simulink model "boostObserver_complete"  (R2020a)
settings: Solver=ode45  StartTime=0.0  StopTime=1.2  FixedStep=0.0005  AbsTol=1e-06  EnableMultiTasking=on
InitFcn:
  | kp=0.01;
  | ki=0.01;
  | 
  | k=2;
  | em=100000000;
  | GE=1/em;
  | GU=k*ki/GE;
  | GCE=k*kp/GU;
model workspace (MAT data in the model file):
  time = 0.8
values from neighbouring files (symbols this model uses):
  AlarmDeadTime = 0.50    (= 0.5)    [BoostFaultSimulation.m]    (also in workspace_atual.mat; workspace_certo.mat)
  B1f = [200 0]    [workspace_atual.mat]    (also in workspace_certo.mat)
  B2f = [200 0]    [workspace_atual.mat]    (also in workspace_certo.mat)
  CiL = [0 1]    [workspace_atual.mat]    (also in workspace_certo.mat)
  CVc = [1 0]    [workspace_atual.mat]    (also in workspace_certo.mat)
  F_11 = -16.4    [workspace_atual.mat]    (also in workspace_certo.mat)
  F_12 = -4812476.87956    [workspace_atual.mat]    (also in workspace_certo.mat)
  F_21 = -3.50877192982    [workspace_atual.mat]    (also in workspace_certo.mat)
  F_22 = -2.00703596657    [workspace_atual.mat]    (also in workspace_certo.mat)
  FaultClass = 0    [BoostFaultSimulation.m]    (also in workspace_atual.mat = 1; workspace_certo.mat = 1)
  iLFaultSwitch = 0    [BoostFaultSimulation.m]    (also in workspace_atual.mat; workspace_certo.mat)
  iLFaultTime = 1.70    (= 1.7)    [BoostFaultSimulation.m]    (also in workspace_atual.mat; workspace_certo.mat)
  L_11 = -176809.798019    [workspace_atual.mat]    (also in workspace_certo.mat)
  L_12 = -66005538231.6    [workspace_atual.mat]    (also in workspace_certo.mat)
  L_21 = 0.0967961040176    [workspace_atual.mat]    (also in workspace_certo.mat)
  L_22 = 350.985265141    [workspace_atual.mat]    (also in workspace_certo.mat)
  Lnew1 = [0.000426144297292  -1.37628182296; -0.636691353583  10000.3869597]    [workspace_atual.mat]    (also in workspace_certo.mat = [0.00144628510103  0.00148492117427; 0.000288596381821  0.00)
  Lnew2 = [0.000454345330516  -0.588943865675; 0.999552025739  4999.94512306]    [workspace_atual.mat]    (also in workspace_certo.mat = [0.00251672143174  0.00251025627081; 6.60131109739e-05  6.53)
  Q_1 = [13715.5123667  1; 1  0]    [workspace_atual.mat]    (also in workspace_certo.mat)
  Q_2 = [1  0; 0.00750867981628  1]    [workspace_atual.mat]    (also in workspace_certo.mat)
  R = 0.1    [boostResults2Latex.m]    (also in workspace_atual.mat = 0.082; workspace_certo.mat = 0.082)
  ReconfigSwitch = 0    [BoostFaultSimulation.m]    (also in workspace_atual.mat; workspace_certo.mat)
  ReconfigTime = 1.707    [BoostFaultSimulation.m]    (also in workspace_atual.mat; workspace_certo.mat)
  SourceAddFactor = 0.10    (= 0.1)    [BoostFaultSimulation.m]    (also in workspace_atual.mat; workspace_certo.mat)
  SourceAddSwitch = 0    [BoostFaultSimulation.m]    (also in workspace_atual.mat; workspace_certo.mat)
  SourceRemoveFactor = 0.10    (= 0.1)    [BoostFaultSimulation.m]    (also in workspace_atual.mat; workspace_certo.mat)
  T_1 = [1 -13715.5123667]    [workspace_atual.mat]    (also in workspace_certo.mat)
  T_2 = [-0.00750867981628 1]    [workspace_atual.mat]    (also in workspace_certo.mat)
  Ts = 0.0001    [workspace_atual.mat]    (also in workspace_certo.mat)
  uf = 190    [workspace_atual.mat]    (also in workspace_certo.mat)
  VcFaultSwitch = 0    [BoostFaultSimulation.m]    (also in workspace_atual.mat; workspace_certo.mat)
  VcFaultTime = 1.70    (= 1.7)    [BoostFaultSimulation.m]    (also in workspace_atual.mat; workspace_certo.mat)
  xe = obj.boostConverter.equilibriumstate(ve)    [BoostController.m]    (also in workspace_atual.mat = [7.62509288104 380]; workspace_certo.mat = [7.62509288104 380])
undefined symbols (not defined in the file or in its folder): MAXnet, MINnet
libraries: PhdLibrary x38, neural x36, dspstat3 x4, powerlib x2, powerlib_meascontrol x2
(part 1 of 3)
settings Model: SimulationMode=accelerator  Creator=d13go  LastModifiedBy=d13go
settings SolverCC: MaxConsecutiveZCs=10000  ZeroCrossAlgorithm=Adaptive  DecoupledContinuousIntegration=on  MinimalZcImpactIntegration=on
settings DataIOCC: SaveFinalState=on  SaveState=on  LoggingToFile=on
settings OptimizationCC: DefaultParameterBehavior=Inlined  UseDivisionForNetSlopeComputation=on  GainParamInheritBuiltInType=on  UseFloatMulNetSlope=on  InlineInvariantSignals=on  EfficientFloat2IntCast=on  LifeSpan=1
settings DebuggingCC: ReadBeforeWriteMsg=DisableAll  WriteAfterWriteMsg=DisableAll  WriteAfterReadMsg=DisableAll  AlgebraicLoopMsg=error  MaxConsecutiveZCsMsg=warning  MaskedZcDiagnostic=none  IgnoredZcDiagnostic=none  MultiTaskDSMMsg=none  SFUnexpectedBacktrackingDiag=warning  SFNoUnconditionalDefaultTransitionDiag=warning  ArithmeticOperatorsInVariantConditions=warning
settings HardwareCC: ProdLongLongMode=on
settings ModelReferenceCC: UpdateModelReferenceTargets=IfOutOfDate
settings SFSimCC: SFSimEcho=off  SimUseLocalCustomCode=off  MATLABDynamicMemAlloc=off  CustomCodeUndefinedFunction=UseInterfaceOnly
settings RTWCC: GenerateReport=on  RTWUseLocalCustomCode=off  LaunchReport=on
settings CodeAppCC: ForceParamTrailComments=on
settings GRTTargetCC: TargetLangStandard=C89/C90 (ANSI)  CombineSignalStateStructs=on  MatFileLogging=off  SupportVariableSizeSignals=on
settings ConfigComp: CovMetricSettings=dw  CovHtmlReporting=on  CovSaveCumulativeToWorkspaceVar=on  CovSaveSingleToWorkspaceVar=on  CovExternalEMLEnable=off
settings SimscapeCC: SimscapeNormalizeSystem=off

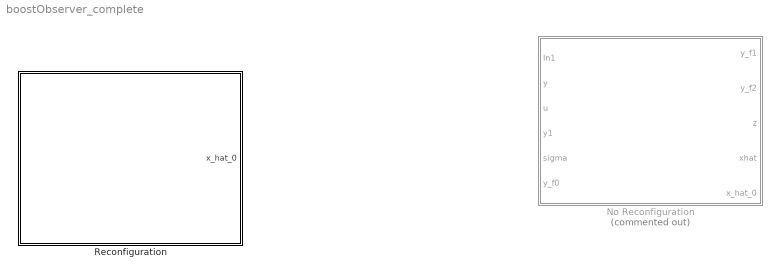
== system boostObserver_complete ==
  No Reconfiguration : Subsystem  Commented=on
  Reconfiguration : Subsystem

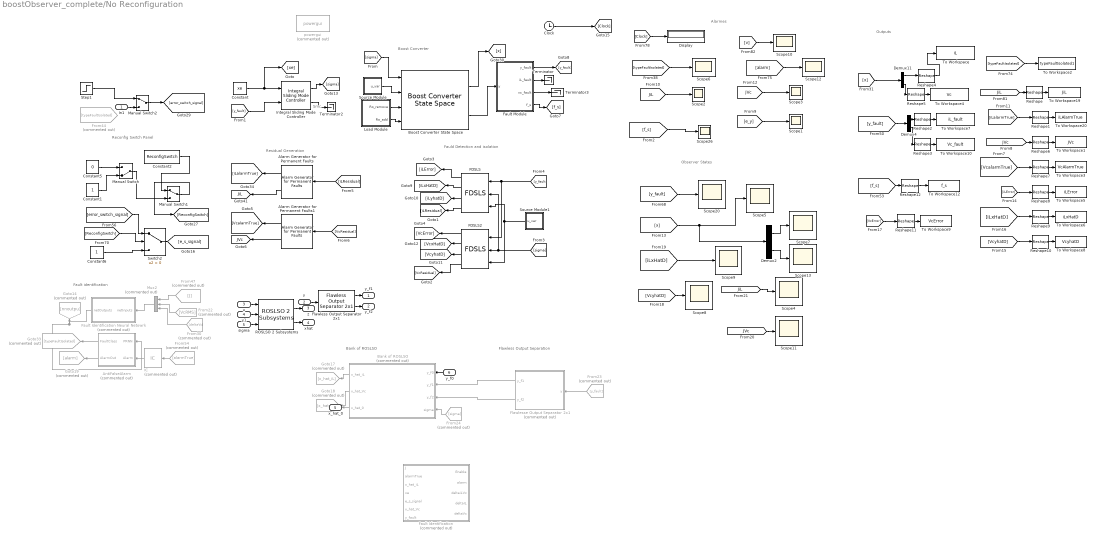
== system boostObserver_complete/No Reconfiguration ==
  note: Fauld Detection and isolation
  note: Smc
  note: Alarmes
  note: Observer States
  note: Residual Generation
  note: Boost Converter
  note: Outputs
  note: Reconfig Switch Panel
  note: Fault identification
  note: Bank of ROSLSO
  note: Flawless Output Separation
  In1 : Inport
  y : Inport  Port=2
  u : Inport  Port=3
  y1 : Inport  Port=4
  sigma : Inport  Port=5
  y_f0 : Inport  Port=6
  Alarm Generator for Permanent Faults : PhdLibrary/Alarm Generator for Permanent Faults  Jth=iLJth  r0=0
      settings: SourceProductName=Phd Diego
  Alarm Generator for Permanent Faults1 : PhdLibrary/Alarm Generator for Permanent Faults  Jth=iLJth  r0=0
      settings: SourceProductName=Phd Diego
  AntiFalseAlarm : Subsystem  Commented=on
  Bank of ROSLSO : Subsystem  Commented=on
  Boost Converter State Space : PhdLibrary/Boost Converter  State Space  A1=A1  A2=A2  B1=B1  R=R  Ro=Ro  Cmatrix=Cmatrix  c=c  LoadAddFactor=LoadAddFactor  LoadRemoveFactor=LoadRemoveFactor
      settings: SourceProductName=Phd Diego
  Clock : Clock
  Constant : Constant  Value=xe  VectorParams1D=off
  Constant1 : Constant
  Constant2 : Constant  Value=ReconfigSwitch
  Constant5 : Constant  Value=0
  Constant6 : Constant
  Demux11 : Demux  Outputs=2
  Demux2 : Demux  Outputs=2
  Demux4 : Demux  Outputs=2
  Display : Display
  FDSLS : PhdLibrary/FDSLS  A1=A1  A2=A2  B1=B1  B2=B2  L=Lnew1  yhat0=[0;0]  x0=[0;0]  Qr=[1 0]
      settings: SourceProductName=Phd Diego
  FDSLS2 : PhdLibrary/FDSLS  A1=A1  A2=A2  B1=B1  B2=B2  L=Lnew2  yhat0=[0;0]  x0=[0;0]  Qr=[0 1]
      settings: SourceProductName=Phd Diego
  Fault Identification : Subsystem  Commented=on
  Fault Identification Neural Netowrk : Subsystem  Commented=on
  Fault Module : Subsystem
  Flawless Output Separator 2x1 : PhdLibrary/Flawless Output  Separator 2x1  Cf1=0  Cf2=0
      settings: SourceProductName=Phd Diego
  Flawlesse Output Separator 2x1 : Subsystem  Commented=on  mask(Flawless Output Separator){Cf1=0, Cf2=0}
      mask prompts: Cf1 "Fault matrix 1"; Cf2 "Fault matrix 2"
      mask help: Separates the 2x1 output
  From22 : From  Commented=on  GotoTag=VcRMS  TagVisibility=global
  From23 : From  Commented=on  GotoTag=y_fault
  From24 : From  Commented=on  GotoTag=sigma
  From30 : From  Commented=on  GotoTag=deltaVc
  From44 : From  Commented=on  GotoTag=typeFaultIsolated
  From47 : From  Commented=on  GotoTag=J  TagVisibility=global
  From54 : From  Commented=on  GotoTag=alarmTrue
  Goto14 : Goto  Commented=on  GotoTag=nnoutpu
  Goto17 : Goto  Commented=on  GotoTag=x_hat_iL
  Goto18 : Goto  Commented=on  GotoTag=x_hat_Vc
  Goto19 : Goto  Commented=on  GotoTag=alarm
  Goto33 : Goto  Commented=on  GotoTag=typeFaultIsolated
  IC : InitialCondition  Commented=on  Value=0
  Integral Sliding Mode Controller : PhdLibrary/Integral Sliding  Mode Controller  KiVc=SmIntegralGain  KVc=SmVcGain  ueq=ueq  Smep=Smep  KiL=SmiLGain  Freq=SmFrequency  x0=0
      settings: SourceProductName=Phd Diego
  Load Module : Subsystem
  Manual Switch : ManualSwitch  CurrentSetting=0
  Manual Switch1 : ManualSwitch
  Manual Switch2 : ManualSwitch
  Mux2 : Mux  Commented=on  Inputs=3
  ROSLSO 2 Subsystems : PhdLibrary/ROSLSO  2 Subsystems  B1=0  B2=0  T=0  F1=0  F2=0  L1=0  L2=0  Q=0  z0=0
      settings: SourceProductName=Phd Diego
  Reshape{,1..12} (13 alike) : Reshape
  Scope{1..13,20,26} (15 alike) : Scope
  Source Module : Subsystem
  Source Module1 : Subsystem
  Step1 : Step  Time=ReconfigTime  After=FaultClass  SampleTime=0
  Switch2 : Switch  Criteria=u2 > Threshold
  Terminator : Terminator
  Terminator2 : Terminator
  Terminator3 : Terminator
  To Workspace : ToWorkspace  VariableName=iL  SaveFormat=Timeseries  SampleTime=-1
  To Workspace1 : ToWorkspace  VariableName=JVc  SaveFormat=Timeseries  SampleTime=-1
  To Workspace10 : ToWorkspace  VariableName=Vc_fault  SaveFormat=Timeseries  SampleTime=-1
  To Workspace12 : ToWorkspace  VariableName=f_s  SaveFormat=Timeseries  SampleTime=-1
  To Workspace19 : ToWorkspace  VariableName=JiL  SaveFormat=Timeseries  SampleTime=-1
  To Workspace2 : ToWorkspace  VariableName=typeFaultIsolated1  SaveFormat=Timeseries  SampleTime=-1
  To Workspace20 : ToWorkspace  VariableName=iLAlarmTrue  SaveFormat=Timeseries  SampleTime=-1
  To Workspace3 : ToWorkspace  VariableName=VcAlarmTrue  SaveFormat=Timeseries  SampleTime=-1
  To Workspace4 : ToWorkspace  VariableName=Vc  SaveFormat=Timeseries  SampleTime=-1
  To Workspace5 : ToWorkspace  VariableName=iLError  SaveFormat=Timeseries  SampleTime=-1
  To Workspace6 : ToWorkspace  VariableName=iLxHatD  SaveFormat=Timeseries  SampleTime=-1
  To Workspace7 : ToWorkspace  VariableName=iL_fault  SaveFormat=Timeseries  SampleTime=-1
  To Workspace8 : ToWorkspace  VariableName=VcyhatD  SaveFormat=Timeseries  SampleTime=-1
  To Workspace9 : ToWorkspace  VariableName=VcError  SaveFormat=Timeseries  SampleTime=-1
  powergui : powerlib/powergui  Priority=1  Commented=on  SimulationMode=Discrete  SampleTime=50e-6  frequency=60  Iterations=50  frequencyindice=0  Pbase=100e6  ErrMax=1e-4  UnitsV=kV  UnitsW=MW  buscounter=0  FunctionMessages=off  echomessages=off  EnableUseOfTLC=off  CurrentSourceSwitches=off  DisableSnubberDevices=off  DisableRonSwitches=off  DisableVfSwitches=off  DisplayEquations=off  AutomaticDiscreteSolvers=off  SolverType=Tustin/Backward Euler (TBE)  Interpol=off  ExternalGateDelay=off  methode=off  Ts=100  x0status=blocks  SPID=on  SwTol=0  HookPort=off  NonlinearTolerance=1e-4  nMaxIteration=100  ContinueOnMaxIteration=off  RestoreLinks=warning  ResistiveCurrentMeasurement=off  Frange=[0:2:500]  Ylog=off  Xlog=on  ShowGrid=off  save=off  variable=ZData  structure=0  ZoomFFT=off  StartTime=0.0  cycles=1  DisplayStyle=1  fundamental=60  FreqAxis=off  MaxFrequency=1000  frequencyindicesteady=1  RmsSteady=1  display=off
  y_f1 : Outport
  y_f2 : Outport  Port=2
  z : Outport  Port=3
  xhat : Outport  Port=4
  x_hat_0 : Outport  Port=5
  tag scope: JVc=global, JiL=global
  wires:
  FDSLS2/1 -> [VcError]
  FDSLS/2 -> [iLxHatD]
  [sigma] -> FDSLS2/2, FDSLS/2
  [iLalarmTrue] -> Reshape1/1
  Reshape11/1 -> To Workspace9/1
  [sigma] -> Boost Converter State Space/1
  Demux2/1 -> Scope7/1
  Reshape9/1 -> To Workspace6/1
  [VcalarmTrue] -> Reshape7/1
  Reshape2/1 -> To Workspace7/1
  [x] -> Demux2/1, Scope5/1
  Load Module/2(Ro_add) -> Boost Converter State Space/4
  Constant/1 -> [xe], Integral Sliding Mode Controller/1
  Constant5/1 -> Manual Switch/1
  [VcyhatD] -> Reshape10/1
  Reshape/1 -> To Workspace19/1
  Reshape4/1 -> To Workspace/1
  Clock/1 -> [Clock]
  [VcResidual] -> Alarm Generator for Permanent Faults1/1
  Alarm Generator for Permanent Faults1/1 -> [VcalarmTrue]
  Reshape10/1 -> To Workspace8/1
  Fault Module/1(y_fault) -> [y_fault]
  [x] -> Demux11/1
  Demux4/1 -> Reshape2/1
  y_f0/1 -> Bank of ROSLSO/1(y_f0)
  Demux11/1 -> Reshape4/1
  FDSLS/4 -> [iLResidual]
  Integral Sliding Mode Controller/2 -> Terminator2/1
  Reshape8/1 -> To Workspace5/1
  Fault Module/3(vc_fault) -> Terminator3/1
  FDSLS/3 -> [iLyhatD]
  Reshape5/1 -> To Workspace4/1
  [JiL] -> Reshape/1
  FDSLS2/4 -> [VcResidual]
  [y_fault] -> Scope20/1
  Boost Converter State Space/2 -> Fault Module/1(y)
  [y_fault] -> FDSLS2/1, FDSLS/1
  [typeFaultIsolated] -> To Workspace2/1
  [f_s] -> Scope26/1
  Reshape1/1 -> To Workspace20/1
  [e_y] -> Scope1/1
  FDSLS2/3 -> [VcyhatD]
  [y_fault] -> Demux4/1
  [error_switch_signal] -> Switch2/1
  [Clock] -> Display/1
  Demux2/2 -> Scope13/1
  Boost Converter State Space/1 -> [x]
  [v] -> Scope10/1
  [JiL] -> Scope2/1
  [JVc] -> Scope3/1
  Alarm Generator for Permanent Faults/2 -> [JiL]
  [alarm] -> Scope12/1
  [VcError] -> Reshape11/1
  Integral Sliding Mode Controller/1 -> [sigma]
  Alarm Generator for Permanent Faults1/2 -> [JVc]
  [iLxHatD] -> Reshape9/1
  [typeFaultIsolated] -> Scope6/1
  [JVc] -> Reshape6/1
  Bank of ROSLSO/3(x_hat_0) -> x_hat_0/1
  [iLResidual] -> Alarm Generator for Permanent Faults/1
  [f_s] -> Reshape12/1
  Load Module/1(Ro_remove) -> Boost Converter State Space/3
  Demux4/2 -> Reshape3/1
  [iLError] -> Reshape8/1
  Step1/1 -> Manual Switch2/1
  FDSLS/1 -> [iLError]
  Reshape6/1 -> To Workspace1/1
  Demux11/2 -> Reshape5/1
  Switch2/1 -> [e_s_signal]
  Alarm Generator for Permanent Faults/1 -> [iLalarmTrue]
  Source Module1/1(u_var) -> FDSLS2/3, FDSLS/3
  [iLxHatD] -> Scope9/1
  Source Module/1(u_var) -> Boost Converter State Space/2
  FDSLS2/2 -> [VcxHatD]
  Fault Module/2(iL_fault) -> Terminator/1
  [JVc] -> Scope11/1
  Reshape3/1 -> To Workspace10/1
  Reshape7/1 -> To Workspace3/1
  Reshape12/1 -> To Workspace12/1
  [JiL] -> Scope4/1
  [VcyhatD] -> Scope8/1
  [y_fault] -> Integral Sliding Mode Controller/2
  Bank of ROSLSO/1(x_hat_iL) -> Goto17/1
  Manual Switch2/1 -> [error_switch_signal]
  Constant1/1 -> Manual Switch/2
  Constant2/1 -> Manual Switch1/1
  Manual Switch/1 -> Manual Switch1/2
  [ReconfigSwitch] -> Switch2/2
  Manual Switch1/1 -> [ReconfigSwitch]
  Constant6/1 -> Switch2/3
  Fault Module/4(f_s) -> [f_s]
  Fault Identification Neural Netowrk/1(netOutputs) -> AntiFalseAlarm/1(PRNN), Goto14/1
  From30/1 -> Mux2/3
  IC/1 -> AntiFalseAlarm/2(Alarm)
  From54/1 -> IC/1
  AntiFalseAlarm/1(FaultClass) -> Goto33/1
  Mux2/1 -> Fault Identification Neural Netowrk/1(netInputs)
  AntiFalseAlarm/2(AlarmOut) -> Goto19/1
  From47/1 -> Mux2/1
  From22/1 -> Mux2/2
  Flawlesse Output Separator 2x1/1(y_f1) -> Bank of ROSLSO/2(y_f1)
  From23/1 -> Flawlesse Output Separator 2x1/1(y)
  Bank of ROSLSO/2(x_hat_Vc) -> Goto18/1
  From24/1 -> Bank of ROSLSO/4(sigma)
  Flawlesse Output Separator 2x1/2(y_f2) -> Bank of ROSLSO/3(y_f2)
  u/1 -> ROSLSO 2 Subsystems/1
  ROSLSO 2 Subsystems/1 -> z/1
  y1/1 -> ROSLSO 2 Subsystems/2
  In1/1 -> Manual Switch2/2
  sigma/1 -> ROSLSO 2 Subsystems/3
  ROSLSO 2 Subsystems/2 -> xhat/1
  Flawless Output Separator 2x1/2 -> y_f2/1
  y/1 -> Flawless Output Separator 2x1/1
  Flawless Output Separator 2x1/1 -> y_f1/1

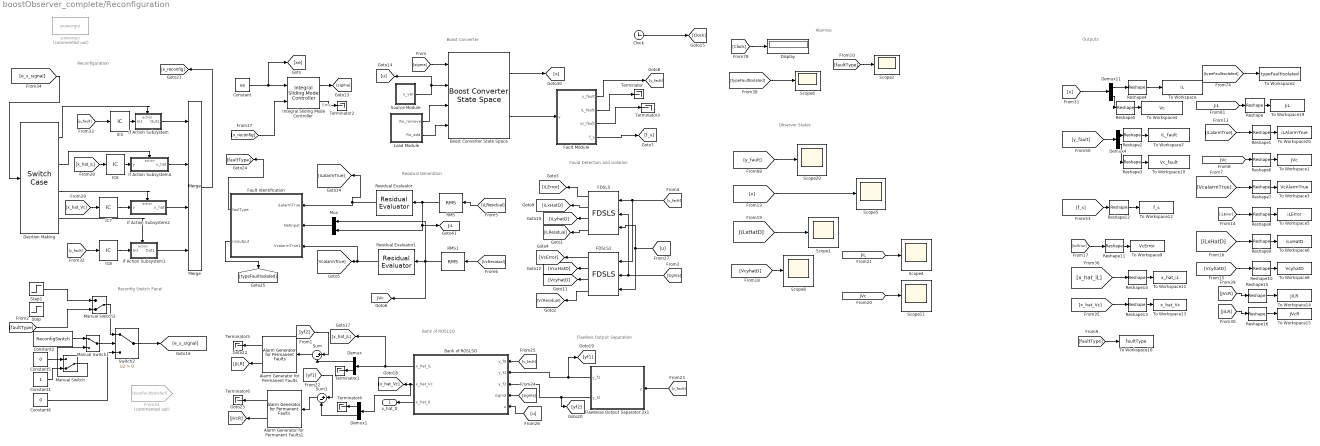
== system boostObserver_complete/Reconfiguration ==
  note: Fauld Detection and isolation
  note: Smc
  note: Alarmes
  note: Observer States
  note: Residual Generation
  note: Boost Converter
  note: Outputs
  note: Bank of ROSLSO
  note: Flawless Output Separation
  note: Reconfiguration
  note: Reconfig Switch Panel
  Alarm Generator for Permanent Faults : PhdLibrary/Alarm Generator for Permanent Faults  Jth=0  r0=0
      settings: SourceProductName=Phd Diego
  Alarm Generator for Permanent Faults1 : PhdLibrary/Alarm Generator for Permanent Faults  Jth=0  r0=0
      settings: SourceProductName=Phd Diego
  Bank of ROSLSO : Subsystem
  Boost Converter State Space : PhdLibrary/Boost Converter  State Space  A1=A1  A2=A2  B1=B1  R=R  Ro=Ro  Cmatrix=Cmatrix  c=c  LoadAddFactor=LoadAddFactor  LoadRemoveFactor=LoadRemoveFactor
      settings: SourceProductName=Phd Diego
  Clock : Clock
  Constant : Constant  Value=xe  VectorParams1D=off
  Constant1 : Constant
  Constant2 : Constant  Value=ReconfigSwitch
  Constant5 : Constant  Value=0
  Constant6 : Constant  Value=0
  Decition Making : SwitchCase  CaseConditions={[0],[1],[2]}
  Demux{,1,4,11} (4 alike) : Demux  Outputs=2
  Display : Display
  FDSLS : PhdLibrary/FDSLS  A1=A1  A2=A2  B1=B1  B2=B2  L=Lnew1  yhat0=[0;0]  x0=[0;0]  Qr=[1 0]
      settings: SourceProductName=Phd Diego
  FDSLS2 : PhdLibrary/FDSLS  A1=A1  A2=A2  B1=B1  B2=B2  L=Lnew2  yhat0=[0;0]  x0=[0;0]  Qr=[0 1]
      settings: SourceProductName=Phd Diego
  Fault Identification : Subsystem
  Fault Module : Subsystem
  Flawlesse Output Separator 2x1 : Subsystem  mask(Flawless Output Separator){Cf1=CiL, Cf2=CVc}
      mask prompts: Cf1 "Fault matrix 1"; Cf2 "Fault matrix 2"
      mask help: Separates the 2x1 output
  From44 : From  Commented=on  GotoTag=typeFaultIsolated
  IC{5..8} (4 alike) : InitialCondition  Value=[0;0]
  If Action Subsystem : Subsystem  TreatAsAtomicUnit=on
  If Action Subsystem1 : Subsystem  TreatAsAtomicUnit=on
  If Action Subsystem2 : Subsystem  TreatAsAtomicUnit=on
  If Action Subsystem4 : Subsystem  TreatAsAtomicUnit=on
  Integral Sliding Mode Controller : PhdLibrary/Integral Sliding  Mode Controller  KiVc=SmIntegralGain  KVc=SmVcGain  ueq=ueq  Smep=Smep  KiL=SmiLGain  Freq=7000  x0=[0;0]  Ts=0
      settings: SourceProductName=Phd Diego
  Load Module : Subsystem
  Manual Switch : ManualSwitch  CurrentSetting=0
  Manual Switch1 : ManualSwitch
  Manual Switch2 : ManualSwitch  CurrentSetting=0
  Merge : Merge  Inputs=4
  Mux : Mux  Inputs=2
  RMS : powerlib_meascontrol/Measurements/RMS  TrueRMS=on  Freq=RMSfrequency  RMSInit=0  Ts=Ts
  RMS1 : powerlib_meascontrol/Measurements/RMS  TrueRMS=on  Freq=RMSfrequency  RMSInit=0  Ts=Ts
  Reshape{,1..16} (17 alike) : Reshape
  Residual Evaluator : PhdLibrary/Residual Evaluator  Jth=iLJth
      settings: SourceProductName=Phd Diego
  Residual Evaluator1 : PhdLibrary/Residual Evaluator  Jth=VcJth
      settings: SourceProductName=Phd Diego
  Scope{1..2,4..6,8,11,20} (8 alike) : Scope
  Source Module : Subsystem
  Step : Step  Time=1.707  After=2  SampleTime=0
  Step1 : Step  Time=ReconfigTime  After=FaultClass  SampleTime=0
  Sum : Sum  Inputs=|+-
  Sum1 : Sum  Inputs=|+-
  Switch2 : Switch  Criteria=u2 > Threshold
  Terminator{,1..6} (7 alike) : Terminator
  To Workspace : ToWorkspace  VariableName=iL  SaveFormat=Timeseries  SampleTime=-1
  To Workspace1 : ToWorkspace  VariableName=JVc  SaveFormat=Timeseries  SampleTime=-1
  To Workspace10 : ToWorkspace  VariableName=Vc_fault  SaveFormat=Timeseries  SampleTime=-1
  To Workspace11 : ToWorkspace  VariableName=x_hat_iL  SaveFormat=Timeseries  SampleTime=-1
  To Workspace12 : ToWorkspace  VariableName=f_s  SaveFormat=Timeseries  SampleTime=-1
  To Workspace13 : ToWorkspace  VariableName=x_hat_Vc  SaveFormat=Timeseries  SampleTime=-1
  To Workspace14 : ToWorkspace  VariableName=JiLR  SaveFormat=Timeseries  SampleTime=-1
  To Workspace15 : ToWorkspace  VariableName=JVcR  SaveFormat=Timeseries  SampleTime=-1
  To Workspace16 : ToWorkspace  VariableName=faultType  SaveFormat=Timeseries  SampleTime=-1
  To Workspace19 : ToWorkspace  VariableName=JiL  SaveFormat=Timeseries  SampleTime=-1
  To Workspace2 : ToWorkspace  VariableName=typeFaultIsolated  SaveFormat=Timeseries  SampleTime=-1
  To Workspace20 : ToWorkspace  VariableName=iLAlarmTrue  SaveFormat=Timeseries  SampleTime=-1
  To Workspace3 : ToWorkspace  VariableName=VcAlarmTrue  SaveFormat=Timeseries  SampleTime=-1
  To Workspace4 : ToWorkspace  VariableName=Vc  SaveFormat=Timeseries  SampleTime=-1
  To Workspace5 : ToWorkspace  VariableName=iLError  SaveFormat=Timeseries  SampleTime=-1
  To Workspace6 : ToWorkspace  VariableName=iLxHatD  SaveFormat=Timeseries  SampleTime=-1
  To Workspace7 : ToWorkspace  VariableName=iL_fault  SaveFormat=Timeseries  SampleTime=-1
  To Workspace8 : ToWorkspace  VariableName=VcyhatD  SaveFormat=Timeseries  SampleTime=-1
  To Workspace9 : ToWorkspace  VariableName=VcError  SaveFormat=Timeseries  SampleTime=-1
  powergui : powerlib/powergui  Priority=1  Commented=on  SimulationMode=Discrete  SampleTime=50e-6  frequency=60  Iterations=50  frequencyindice=0  Pbase=100e6  ErrMax=1e-4  UnitsV=kV  UnitsW=MW  buscounter=0  FunctionMessages=off  echomessages=off  EnableUseOfTLC=off  CurrentSourceSwitches=off  DisableSnubberDevices=off  DisableRonSwitches=off  DisableVfSwitches=off  DisplayEquations=off  AutomaticDiscreteSolvers=off  SolverType=Tustin/Backward Euler (TBE)  Interpol=off  ExternalGateDelay=off  methode=off  Ts=100  x0status=blocks  SPID=on  SwTol=0  HookPort=off  NonlinearTolerance=1e-4  nMaxIteration=100  ContinueOnMaxIteration=off  RestoreLinks=warning  ResistiveCurrentMeasurement=off  Frange=[0:2:500]  Ylog=off  Xlog=on  ShowGrid=off  save=off  variable=ZData  structure=0  ZoomFFT=off  StartTime=0.0  cycles=1  DisplayStyle=1  fundamental=60  FreqAxis=off  MaxFrequency=1000  frequencyindicesteady=1  RmsSteady=1  display=off
  x_hat_0 : Outport
  tag scope: JVc=global, JiL=global
  wires:
  FDSLS2/1 -> [VcError]
  FDSLS/2 -> [iLxHatD]
  [sigma] -> FDSLS2/2, FDSLS/2
  [iLalarmTrue] -> Reshape1/1
  Reshape11/1 -> To Workspace9/1
  [sigma] -> Boost Converter State Space/1
  Reshape9/1 -> To Workspace6/1
  [VcalarmTrue] -> Reshape7/1
  Reshape2/1 -> To Workspace7/1
  [x] -> Scope5/1
  Constant/1 -> Integral Sliding Mode Controller/1, [xe]
  [VcyhatD] -> Reshape10/1
  Reshape/1 -> To Workspace19/1
  Reshape4/1 -> To Workspace/1
  Clock/1 -> [Clock]
  Residual Evaluator1/1 -> Fault Identification/3(VcalarmTrue1), [VcalarmTrue]
  Reshape10/1 -> To Workspace8/1
  Fault Module/1(y_fault) -> [y_fault]
  [x] -> Demux11/1
  Demux4/1 -> Reshape2/1
  [y_fault] -> Bank of ROSLSO/1(y_f0)
  Demux11/1 -> Reshape4/1
  FDSLS/4 -> [iLResidual]
  Integral Sliding Mode Controller/2 -> Terminator2/1
  Reshape8/1 -> To Workspace5/1
  Fault Module/3(vc_fault) -> Terminator3/1
  FDSLS/3 -> [iLyhatD]
  Reshape5/1 -> To Workspace4/1
  [JiL] -> Reshape/1
  FDSLS2/4 -> [VcResidual]
  [y_fault] -> Scope20/1
  Boost Converter State Space/2 -> Fault Module/1(y)
  [y_fault] -> FDSLS2/1, FDSLS/1
  [typeFaultIsolated] -> To Workspace2/1
  Reshape1/1 -> To Workspace20/1
  FDSLS2/3 -> [VcyhatD]
  [y_fault] -> Demux4/1
  [Clock] -> Display/1
  Boost Converter State Space/1 -> [x]
  [VcError] -> Reshape11/1
  Integral Sliding Mode Controller/1 -> [sigma]
  [iLxHatD] -> Reshape9/1
  [typeFaultIsolated] -> Scope6/1
  [JVc] -> Reshape6/1
  Bank of ROSLSO/3(x_hat_0) -> x_hat_0/1
  [f_s] -> Reshape12/1
  Demux4/2 -> Reshape3/1
  [iLError] -> Reshape8/1
  FDSLS/1 -> [iLError]
  Reshape6/1 -> To Workspace1/1
  Demux11/2 -> Reshape5/1
  Residual Evaluator/1 -> Fault Identification/1(iLalarmTrue), [iLalarmTrue]
  [u] -> FDSLS/3, FDSLS2/3
  [iLxHatD] -> Scope1/1
  FDSLS2/2 -> [VcxHatD]
  Fault Module/2(iL_fault) -> Terminator/1
  [JVc] -> Scope11/1
  Reshape3/1 -> To Workspace10/1
  Reshape7/1 -> To Workspace3/1
  Reshape12/1 -> To Workspace12/1
  [VcyhatD] -> Scope8/1
  Bank of ROSLSO/1(x_hat_iL) -> [x_hat_iL], Demux/1
  Fault Module/4(f_s) -> [f_s]
  [y_fault] -> Flawlesse Output Separator 2x1/1(y)
  [sigma] -> Bank of ROSLSO/4(sigma)
  Flawlesse Output Separator 2x1/2(y_f2) -> [yf2], Bank of ROSLSO/3(y_f2)
  [u] -> Bank of ROSLSO/5(u)
  [x_hat_Vc] -> IC7/1
  [e_s_signal] -> Decition Making/1
  If Action Subsystem2/1(x_hat) -> Merge/3
  IC8/1 -> If Action Subsystem1/1(In1)
  IC6/1 -> If Action Subsystem4/1(y)
  [x_hat_iL] -> IC6/1
  Merge/1 -> [x_reconfig]
  IC5/1 -> If Action Subsystem/1(In1)
  If Action Subsystem1/1(Out1) -> Merge/4
  Decition Making/2 -> If Action Subsystem4/Action
  Decition Making/1 -> If Action Subsystem/Action
  Decition Making/3 -> If Action Subsystem2/Action
  IC7/1 -> If Action Subsystem2/1(y)
  [y_fault] -> IC5/1
  Decition Making/4 -> If Action Subsystem1/Action
  If Action Subsystem4/1(x_hat) -> Merge/2
  [y_fault] -> IC8/1
  If Action Subsystem/1(Out1) -> Merge/1
  [x_hat_iL] -> Reshape14/1
  Reshape13/1 -> To Workspace13/1
  [x_hat_Vc] -> Reshape13/1
  Reshape14/1 -> To Workspace11/1
  Step1/1 -> Manual Switch2/1
  Manual Switch/1 -> Manual Switch1/2
  Constant2/1 -> Manual Switch1/1
  Constant1/1 -> Manual Switch/2
  Constant5/1 -> Manual Switch/1
  Manual Switch1/1 -> Switch2/2
  Constant6/1 -> Switch2/3
  Manual Switch2/1 -> Switch2/1
  Switch2/1 -> [e_s_signal]
  Source Module/1(u_var) -> Boost Converter State Space/2, [u]
  Bank of ROSLSO/2(x_hat_Vc) -> Demux1/1, [x_hat_Vc]
  Flawlesse Output Separator 2x1/1(y_f1) -> [yf1], Bank of ROSLSO/2(y_f1)
  [yf2] -> Sum/1
  Alarm Generator for Permanent Faults/2 -> [JiLR]
  Demux/1 -> Sum/2
  [yf1] -> Sum1/1
  Demux1/2 -> Sum1/2
  Sum1/1 -> Alarm Generator for Permanent Faults1/1
  [JVcR] -> Reshape15/1
  [JiLR] -> Reshape16/1
  Reshape15/1 -> To Workspace14/1
  Reshape16/1 -> To Workspace15/1
  [JiL] -> Scope4/1
  Alarm Generator for Permanent Faults1/2 -> [JVcR]
  Sum/1 -> Alarm Generator for Permanent Faults/1
  Demux/2 -> Terminator1/1
  Demux1/1 -> Terminator4/1
  Alarm Generator for Permanent Faults/1 -> Terminator5/1
  Alarm Generator for Permanent Faults1/1 -> Terminator6/1
  [x_reconfig] -> Integral Sliding Mode Controller/2
  RMS/1 -> [JiL], Mux/2, Residual Evaluator/1
  [VcResidual] -> RMS1/1
  Load Module/2(Ro_add) -> Boost Converter State Space/4
  Load Module/1(Ro_remove) -> Boost Converter State Space/3
  Mux/1 -> Fault Identification/2(Netinput)
  Fault Identification/1(faulType) -> [faultType]
  Fault Identification/2(nnoutput) -> [typeFaultIsolated]
  [faultType] -> Manual Switch2/2
  [faultType] -> To Workspace16/1
  [faultType] -> Scope2/1
  [iLResidual] -> RMS/1
  RMS1/1 -> Mux/1, [JVc], Residual Evaluator1/1

== system boostObserver_complete/No Reconfiguration/AntiFalseAlarm ==
  PRNN : Inport
  Alarm : Inport  Port=2
  Constant7 : Constant
  FaultDetecition1 : Switch  Criteria=u2 > Threshold
  Product1 : Product
  Step1 : Step  Time=AlarmDeadTime  SampleTime=0
  FaultClass : Outport
  AlarmOut : Outport  Port=2
  wires:
  PRNN/1 -> FaultDetecition1/1
  Constant7/1 -> FaultDetecition1/3
  Step1/1 -> Product1/1
  Alarm/1 -> Product1/2
  FaultDetecition1/1 -> FaultClass/1
  Product1/1 -> AlarmOut/1, FaultDetecition1/2

== system boostObserver_complete/No Reconfiguration/Bank of ROSLSO ==
  y_f0 : Inport
  y_f1 : Inport  Port=2
  y_f2 : Inport  Port=3
  sigma : Inport  Port=4
  Constant : Constant  Value=uf  VectorParams1D=off
  ROSLSO 2 Subsystems : Subsystem  mask(ROSLSO){B1=B1f, B2=B2f, T=T_1, F1=F_11, F2=F_12, L1=L_11, L2=L_12, Q=Q_1, z0=0}
      mask prompts: B1 "Input matrix system 1:"; B2 "Input matrix system 2:"; T "Input gain matrix:"; F1 "Observer matrix system 1:"; F2 "Observer matrix system 2:"; L1 "Output gain matrix system 1:"; L2 "Output gain matrix system 2:"; Q "Weight matrix"; z0 "Initial conditions:"
      mask help:
      | Reduced Order Switched Linear Systems Observer
      | Estimates only the unmensured variables and concatenate with output
  ROSLSO 2 Subsystems1 : Subsystem  mask(ROSLSO){B1=B1f, B2=B2f, T=T_2, F1=F_21, F2=F_22, L1=L_21, L2=L_22, Q=Q_2, z0=0}
      mask prompts: B1 "Input matrix system 1:"; B2 "Input matrix system 2:"; T "Input gain matrix:"; F1 "Observer matrix system 1:"; F2 "Observer matrix system 2:"; L1 "Output gain matrix system 1:"; L2 "Output gain matrix system 2:"; Q "Weight matrix"; z0 "Initial conditions:"
      mask help:
      | Reduced Order Switched Linear Systems Observer
      | Estimates only the unmensured variables and concatenate with output
  Terminator : Terminator
  Terminator1 : Terminator
  x_hat_iL : Outport
  x_hat_Vc : Outport  Port=2
  x_hat_0 : Outport  Port=3
  wires:
  sigma/1 -> ROSLSO 2 Subsystems/3(sigma), ROSLSO 2 Subsystems1/3(sigma)
  y_f1/1 -> ROSLSO 2 Subsystems/2(y)
  y_f2/1 -> ROSLSO 2 Subsystems1/2(y)
  Constant/1 -> ROSLSO 2 Subsystems/1(u), ROSLSO 2 Subsystems1/1(u)
  ROSLSO 2 Subsystems1/2(xhat) -> x_hat_Vc/1
  ROSLSO 2 Subsystems/2(xhat) -> x_hat_iL/1
  ROSLSO 2 Subsystems/1(z) -> Terminator/1
  ROSLSO 2 Subsystems1/1(z) -> Terminator1/1
  y_f0/1 -> x_hat_0/1

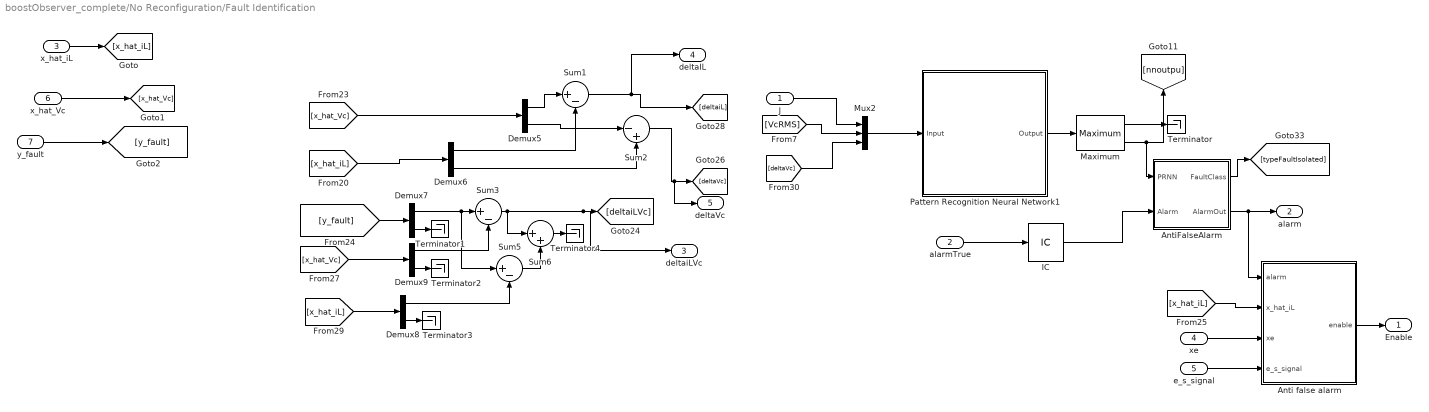
== system boostObserver_complete/No Reconfiguration/Fault Identification ==
  J : Inport
  alarmTrue : Inport  Port=2
  x_hat_iL : Inport  Port=3
  xe : Inport  Port=4
  e_s_signal : Inport  Port=5
  x_hat_Vc : Inport  Port=6
  y_fault : Inport  Port=7
  Anti false alarm : Subsystem
  AntiFalseAlarm : Subsystem
  Demux{5..9} (5 alike) : Demux  Outputs=2
  IC : InitialCondition  Value=0
  Maximum : dspstat3/Maximum  operation=maximum  fcn=Value and Index  indexBase=One  operateOver=Each column  Dimension=1  InputProcessing=Columns as channels (frame based)  reset=None  roiEnable=off  roiType=Rectangles  roiPortion=Entire ROI  roiOutput=Individual statistics for each ROI  roiFlag=off  roundingMode=Floor  overflowMode=off  accumDataTypeStr=Inherit: Same as product output  accumLastDataTypeStr=Inherit: Same as product output
  Mux2 : Mux  Inputs=3
  Pattern Recognition Neural Network1 : Subsystem
      mask help: Pattern Recognition Neural Network
      mask Display: e = 0.06;c1 = [120 150 230]/255;c2 = ([120 150 230]+0)/383;c3 = ([120 150 230]+128)/383;patch([0 1 1 0],[0 0 1 1],c1);patch([0 1 1 1-e 1-e 0+e],[0 0 1 1-e 0+e 0+e],c2);patch([0 0 1 1-e 0+e 0+e],[0 1 1 1-e 1-e 0+e],c3);plot([0 1 1 0 0],[0 0 1 1 0]);fprintf('NNET');port_label('input',1,' Input');port_label('output',1,'Output ');
  Sum1 : Sum  Inputs=|+-
  Sum2 : Sum  Inputs=|-+
  Sum3 : Sum  Inputs=|+-
  Sum5 : Sum  Inputs=|+-
  Sum6 : Sum  Inputs=|++
  Terminator{,1..4} (5 alike) : Terminator
  Enable : Outport
  alarm : Outport  Port=2
  deltaiLVc : Outport  Port=3
  deltaIL : Outport  Port=4
  deltaVc : Outport  Port=5
  wires:
  Demux6/2 -> Sum2/2
  Sum2/1 -> deltaVc/1, [deltaVc]
  Demux7/2 -> Terminator1/1
  Sum5/1 -> Sum6/2
  [y_fault] -> Demux7/1
  Sum3/1 -> deltaiLVc/1, [deltaiLVc], Sum6/1
  Demux5/2 -> Sum2/1
  [x_hat_Vc] -> Demux9/1
  Demux5/1 -> Sum1/1
  Demux9/1 -> Sum3/2
  [deltaVc] -> Mux2/3
  [x_hat_Vc] -> Demux5/1
  Demux6/1 -> Sum1/2
  Demux8/1 -> Sum5/2
  Demux7/1 -> Sum5/1, Sum3/1
  [VcRMS] -> Mux2/2
  [x_hat_iL] -> Demux6/1
  Sum1/1 -> deltaIL/1, [deltaiL]
  [x_hat_iL] -> Demux8/1
  Demux9/2 -> Terminator2/1
  Demux8/2 -> Terminator3/1
  J/1 -> Mux2/1
  Maximum/1 -> Terminator/1
  Pattern Recognition Neural Network1/1(Output) -> Maximum/1
  Mux2/1 -> Pattern Recognition Neural Network1/1(Input)
  Maximum/2 -> AntiFalseAlarm/1(PRNN), [nnoutpu]
  alarmTrue/1 -> IC/1
  IC/1 -> AntiFalseAlarm/2(Alarm)
  AntiFalseAlarm/1(FaultClass) -> [typeFaultIsolated]
  AntiFalseAlarm/2(AlarmOut) -> alarm/1, Anti false alarm/1(alarm)
  xe/1 -> Anti false alarm/3(xe)
  e_s_signal/1 -> Anti false alarm/4(e_s_signal)
  Anti false alarm/1(enable) -> Enable/1
  x_hat_iL/1 -> [x_hat_iL]
  [x_hat_iL] -> Anti false alarm/2(x_hat_iL)
  x_hat_Vc/1 -> [x_hat_Vc]
  y_fault/1 -> [y_fault]
  Sum6/1 -> Terminator4/1

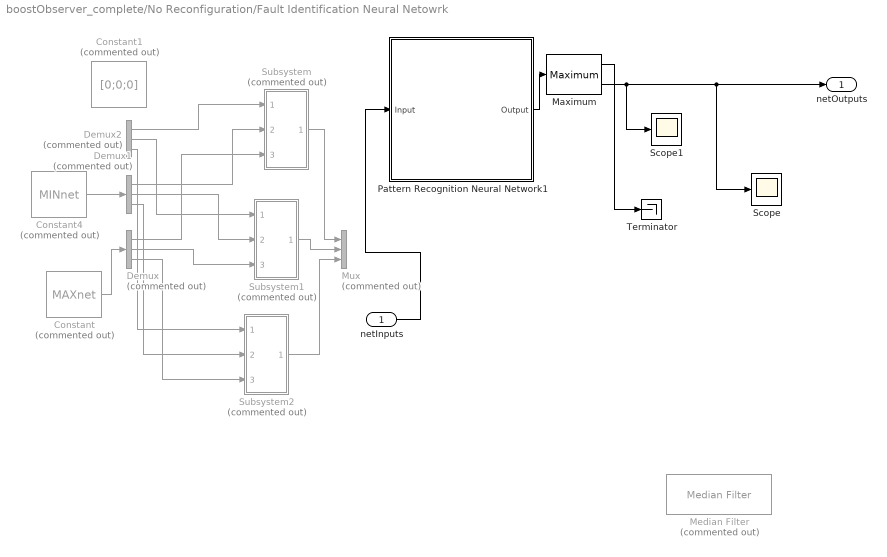
== system boostObserver_complete/No Reconfiguration/Fault Identification Neural Netowrk ==
  netInputs : Inport
  Constant : Constant  Commented=on  Value=MAXnet
  Constant1 : Constant  Commented=on  Value=[0;0;0]
  Constant4 : Constant  Commented=on  Value=MINnet
  Demux : Demux  Commented=on  Outputs=3
  Demux1 : Demux  Commented=on  Outputs=3
  Demux2 : Demux  Commented=on  Outputs=3
  Maximum : dspstat3/Maximum  operation=maximum  fcn=Value and Index  indexBase=One  operateOver=Each column  Dimension=1  InputProcessing=Columns as channels (frame based)  reset=None  roiEnable=off  roiType=Rectangles  roiPortion=Entire ROI  roiOutput=Individual statistics for each ROI  roiFlag=off  roundingMode=Floor  overflowMode=off  accumDataTypeStr=Inherit: Same as product output  accumLastDataTypeStr=Inherit: Same as product output
  Median Filter : dspstat3/Median Filter  Commented=on  WindowLength=1  SimulateUsing=Code generation
      settings: SourceProductBaseCode=DS
  Mux : Mux  Commented=on  Inputs=3
  Pattern Recognition Neural Network1 : Subsystem
      mask help: Pattern Recognition Neural Network
      mask Display: e = 0.06;c1 = [120 150 230]/255;c2 = ([120 150 230]+0)/383;c3 = ([120 150 230]+128)/383;patch([0 1 1 0],[0 0 1 1],c1);patch([0 1 1 1-e 1-e 0+e],[0 0 1 1-e 0+e 0+e],c2);patch([0 0 1 1-e 0+e 0+e],[0 1 1 1-e 1-e 0+e],c3);plot([0 1 1 0 0],[0 0 1 1 0]);fprintf('NNET');port_label('input',1,' Input');port_label('output',1,'Output ');
  Scope : Scope
  Scope1 : Scope
  Subsystem : Subsystem  Commented=on
  Subsystem1 : Subsystem  Commented=on
  Subsystem2 : Subsystem  Commented=on
  Terminator : Terminator
  netOutputs : Outport
  wires:
  Maximum/1 -> Terminator/1
  Maximum/2 -> Scope1/1, netOutputs/1, Scope/1
  Constant/1 -> Demux/1
  Demux2/1 -> Subsystem/1(input)
  Demux1/1 -> Subsystem/2(min)
  Demux/1 -> Subsystem/3(max)
  Demux1/2 -> Subsystem1/2(min)
  Demux/2 -> Subsystem1/3(max)
  Demux2/2 -> Subsystem1/1(input)
  Demux/3 -> Subsystem2/3(max)
  Demux1/3 -> Subsystem2/2(min)
  Demux2/3 -> Subsystem2/1(input)
  Subsystem/1(Out1) -> Mux/1
  Subsystem1/1(Out1) -> Mux/2
  Subsystem2/1(Out1) -> Mux/3
  Constant4/1 -> Demux1/1
  netInputs/1 -> Pattern Recognition Neural Network1/1(Input)
  Pattern Recognition Neural Network1/1(Output) -> Maximum/1

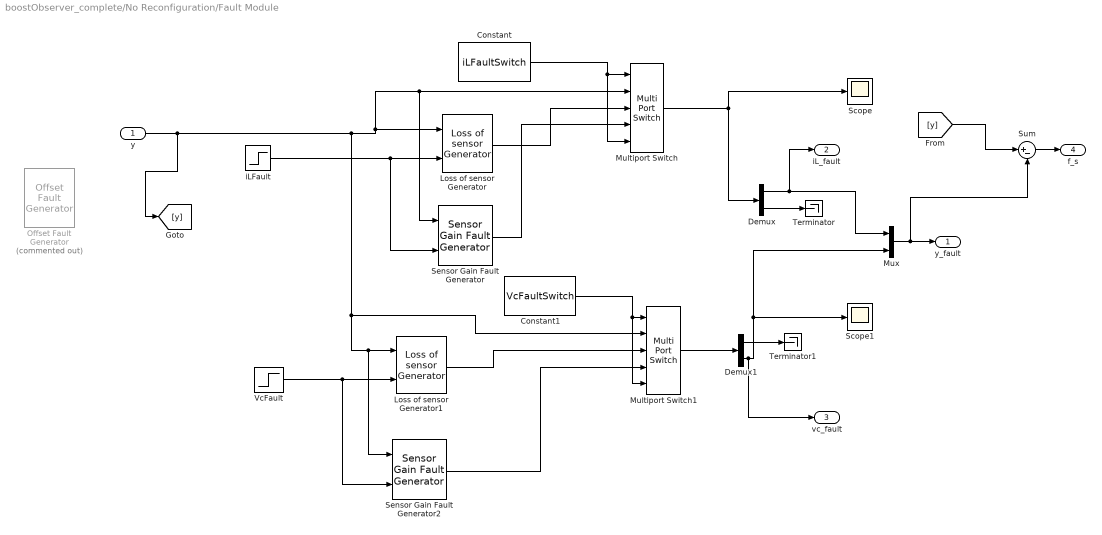
== system boostObserver_complete/No Reconfiguration/Fault Module ==
  y : Inport
  Constant : Constant  Value=iLFaultSwitch
  Constant1 : Constant  Value=VcFaultSwitch
  Demux : Demux  Outputs=2
  Demux1 : Demux  Outputs=2
  Loss of sensor Generator : PhdLibrary/Loss of sensor Generator
      settings: SourceProductName=Phd Diego
  Loss of sensor Generator1 : PhdLibrary/Loss of sensor Generator
      settings: SourceProductName=Phd Diego
  Multiport Switch : MultiPortSwitch  DataPortOrder=Zero-based contiguous  DataPortForDefault=Additional data port  zeroidx=on
  Multiport Switch1 : MultiPortSwitch  DataPortOrder=Zero-based contiguous  DataPortForDefault=Additional data port  zeroidx=on
  Mux : Mux  Inputs=2
  Offset Fault Generator : PhdLibrary/Offset Fault Generator  Commented=on  s1gain=20  s2gain=20
      settings: SourceProductName=Phd Diego
  Scope : Scope
  Scope1 : Scope
  Sensor Gain Fault Generator : PhdLibrary/Sensor Gain Fault Generator  s1gain=iLGainFaultFactor  s2gain=VcGainFaultFactor
      settings: SourceProductName=Phd Diego
  Sensor Gain Fault Generator2 : PhdLibrary/Sensor Gain Fault Generator  s1gain=iLGainFaultFactor  s2gain=VcGainFaultFactor
      settings: SourceProductName=Phd Diego
  Sum : Sum  Inputs=|+-
  Terminator : Terminator
  Terminator1 : Terminator
  VcFault : Step  Time=VcFaultTime  After=2  SampleTime=0
  iLFault : Step  Time=iLFaultTime  SampleTime=0
  y_fault : Outport
  iL_fault : Outport  Port=2
  vc_fault : Outport  Port=3
  f_s : Outport  Port=4
  wires:
  iLFault/1 -> Sensor Gain Fault Generator/2, Loss of sensor Generator/2
  y/1 -> [y], Multiport Switch1/2, Sensor Gain Fault Generator2/1, Loss of sensor Generator1/1, Sensor Gain Fault Generator/1, Multiport Switch/2, Loss of sensor Generator/1
  VcFault/1 -> Sensor Gain Fault Generator2/2, Loss of sensor Generator1/2
  Constant/1 -> Multiport Switch/5, Multiport Switch/1
  Constant1/1 -> Multiport Switch1/5, Multiport Switch1/1
  Multiport Switch/1 -> Demux/1, Scope/1
  Multiport Switch1/1 -> Demux1/1
  Demux/2 -> Terminator/1
  Demux/1 -> iL_fault/1, Mux/1
  Mux/1 -> Sum/2, y_fault/1
  Demux1/1 -> Terminator1/1
  Demux1/2 -> vc_fault/1, Mux/2, Scope1/1
  Loss of sensor Generator/1 -> Multiport Switch/3
  Sensor Gain Fault Generator/1 -> Multiport Switch/4
  Sensor Gain Fault Generator2/1 -> Multiport Switch1/4
  Loss of sensor Generator1/1 -> Multiport Switch1/3
  [y] -> Sum/1
  Sum/1 -> f_s/1

== system boostObserver_complete/No Reconfiguration/Flawlesse Output Separator 2x1 ==
  y : Inport
  Matrizes A1 : Constant  Value=Cf2  VectorParams1D=off
  Matrizes A2 : Constant  Value=Cf1  VectorParams1D=off
  Product : Product  Multiplication=Matrix(*)
  Product1 : Product  Multiplication=Matrix(*)
  y_f1 : Outport
  y_f2 : Outport  Port=2
  wires:
  y/1 -> Product1/2, Product/2
  Matrizes A2/1 -> Product/1
  Matrizes A1/1 -> Product1/1
  Product/1 -> y_f1/1
  Product1/1 -> y_f2/1

== system boostObserver_complete/No Reconfiguration/Load Module ==
  Load_add_switch : PhdLibrary/Step Perturbation  SignalSwitch=LoadAddSignalSwitch  InitialMagnitude=0  InitialTime=LoadAddTime  Magnitude=1  Duration=0  enabled=LoadAddSwitch
      settings: SourceProductName=Phd Diego
  Load_remove_switch : PhdLibrary/Step Perturbation  SignalSwitch=LoadRemoveSignalSwitch  InitialMagnitude=0  InitialTime=LoadRemoveTime  Magnitude=1  Duration=0  enabled=LoadRemoveSwitch
      settings: SourceProductName=Phd Diego
  Ro_remove : Outport
  Ro_add : Outport  Port=2
  wires:
  Load_remove_switch/1 -> Ro_remove/1
  Load_add_switch/1 -> Ro_add/1

== system boostObserver_complete/No Reconfiguration/Source Module ==
  Constant1 : Constant  Value=SourceAddSwitch  VectorParams1D=off
  Constant11 : Constant  Value=u
  Source_add_switch : PhdLibrary/Step Perturbation  SignalSwitch=SourceAddSignalSwitch  InitialMagnitude=u  InitialTime=SourceAddTime  Magnitude=SourceAddFactor*u  Duration=0  enabled=SourceAddSwitch
      settings: SourceProductName=Phd Diego
  Source_remove_switch : PhdLibrary/Step Perturbation  SignalSwitch=SourceRemoveSwitch  InitialMagnitude=u  InitialTime=SourceRemoveTime  Magnitude=-SourceRemoveFactor*u  Duration=0  enabled=SourceRemoveSwitch
      settings: SourceProductName=Phd Diego
  Sum : Sum  Inputs=|++
  Sum1 : Sum  Inputs=|++
  Switch : Switch  Criteria=u2 > Threshold
  u_var : Outport
  wires:
  Sum1/1 -> Switch/3
  Sum/1 -> Switch/1
  Constant11/1 -> Sum1/1, Sum/1
  Switch/1 -> u_var/1
  Source_add_switch/1 -> Sum/2
  Source_remove_switch/1 -> Sum1/2
  Constant1/1 -> Switch/2

== system boostObserver_complete/No Reconfiguration/Source Module1 ==
  Constant1 : Constant  Value=SourceAddSwitch  VectorParams1D=off
  Constant11 : Constant  Value=u
  Source_add_switch : PhdLibrary/Step Perturbation  SignalSwitch=SourceAddSignalSwitch  InitialMagnitude=u  InitialTime=SourceAddTime  Magnitude=SourceAddFactor*u  Duration=0  enabled=SourceAddSwitch
      settings: SourceProductName=Phd Diego
  Source_remove_switch : PhdLibrary/Step Perturbation  SignalSwitch=SourceRemoveSwitch  InitialMagnitude=u  InitialTime=SourceRemoveTime  Magnitude=-SourceRemoveFactor*u  Duration=0  enabled=SourceRemoveSwitch
      settings: SourceProductName=Phd Diego
  Sum : Sum  Inputs=|++
  Sum1 : Sum  Inputs=|++
  Switch : Switch  Criteria=u2 > Threshold
  u_var : Outport
  wires:
  Sum1/1 -> Switch/3
  Sum/1 -> Switch/1
  Constant11/1 -> Sum1/1, Sum/1
  Switch/1 -> u_var/1
  Source_add_switch/1 -> Sum/2
  Source_remove_switch/1 -> Sum1/2
  Constant1/1 -> Switch/2

== system boostObserver_complete/Reconfiguration/Bank of ROSLSO ==
  y_f0 : Inport
  y_f1 : Inport  Port=2
  y_f2 : Inport  Port=3
  sigma : Inport  Port=4
  u : Inport  Port=5
  ROSLSO 2 Subsystems : PhdLibrary/ROSLSO  2 Subsystems  B1=B1f  B2=B2f  T=T_1  F1=F_11  F2=F_12  L1=L_11  L2=L_12  Q=Q_1  z0=0
      settings: SourceProductName=Phd Diego
  ROSLSO 2 Subsystems1 : PhdLibrary/ROSLSO  2 Subsystems  B1=B1f  B2=B2f  T=T_2  F1=F_21  F2=F_22  L1=L_21  L2=L_22  Q=Q_2  z0=0
      settings: SourceProductName=Phd Diego
  Terminator : Terminator
  Terminator1 : Terminator
  x_hat_iL : Outport
  x_hat_Vc : Outport  Port=2
  x_hat_0 : Outport  Port=3
  wires:
  sigma/1 -> ROSLSO 2 Subsystems/3, ROSLSO 2 Subsystems1/3
  y_f1/1 -> ROSLSO 2 Subsystems/2
  y_f2/1 -> ROSLSO 2 Subsystems1/2
  ROSLSO 2 Subsystems1/2 -> x_hat_Vc/1
  ROSLSO 2 Subsystems/2 -> x_hat_iL/1
  ROSLSO 2 Subsystems/1 -> Terminator/1
  ROSLSO 2 Subsystems1/1 -> Terminator1/1
  y_f0/1 -> x_hat_0/1
  u/1 -> ROSLSO 2 Subsystems1/1, ROSLSO 2 Subsystems/1

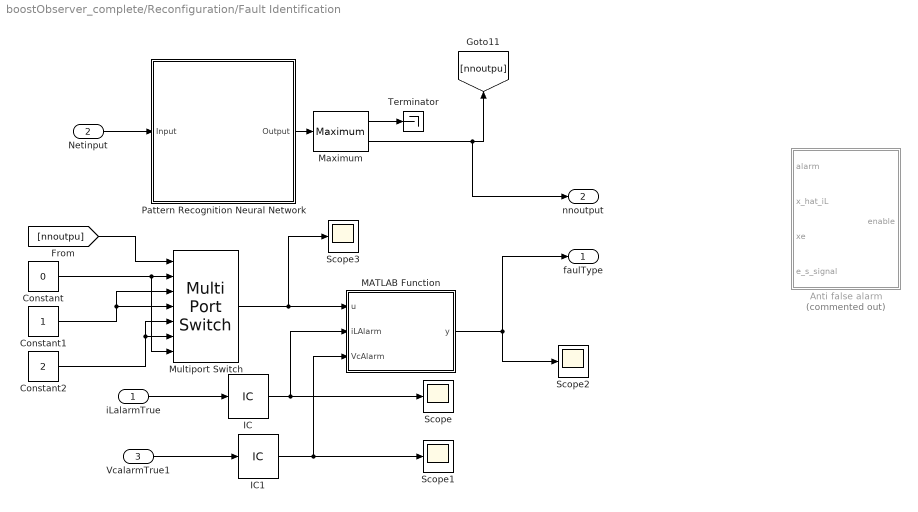
== system boostObserver_complete/Reconfiguration/Fault Identification ==
  iLalarmTrue : Inport
  Netinput : Inport  Port=2
  VcalarmTrue1 : Inport  Port=3
  Anti false alarm : Subsystem  Commented=on
  Constant : Constant  Value=0
  Constant1 : Constant
  Constant2 : Constant  Value=2
  IC : InitialCondition  Value=0
  IC1 : InitialCondition  Value=0
  MATLAB Function : MATLAB Function  TreatAsAtomicUnit=on
  Maximum : dspstat3/Maximum  operation=maximum  fcn=Value and Index  indexBase=One  operateOver=Each column  Dimension=1  InputProcessing=Columns as channels (frame based)  reset=None  roiEnable=off  roiType=Rectangles  roiPortion=Entire ROI  roiOutput=Individual statistics for each ROI  roiFlag=off  roundingMode=Floor  overflowMode=off  accumDataTypeStr=Inherit: Same as product output  accumLastDataTypeStr=Inherit: Same as product output
  Multiport Switch : MultiPortSwitch  Inputs=5  DataPortForDefault=Additional data port
  Pattern Recognition Neural Network : Subsystem
      mask help: Pattern Recognition Neural Network
      mask Display: e = 0.06;c1 = [120 150 230]/255;c2 = ([120 150 230]+0)/383;c3 = ([120 150 230]+128)/383;patch([0 1 1 0],[0 0 1 1],c1);patch([0 1 1 1-e 1-e 0+e],[0 0 1 1-e 0+e 0+e],c2);patch([0 0 1 1-e 0+e 0+e],[0 1 1 1-e 1-e 0+e],c3);plot([0 1 1 0 0],[0 0 1 1 0]);fprintf('NNET');port_label('input',1,' Input');port_label('output',1,'Output ');
  Scope{,1..3} (4 alike) : Scope
  Terminator : Terminator
  faulType : Outport
  nnoutput : Outport  Port=2
  wires:
  Maximum/1 -> Terminator/1
  Pattern Recognition Neural Network/1(Output) -> Maximum/1
  Maximum/2 -> nnoutput/1, [nnoutpu]
  Constant/1 -> Multiport Switch/7, Multiport Switch/2
  Constant1/1 -> Multiport Switch/4, Multiport Switch/3
  Constant2/1 -> Multiport Switch/6, Multiport Switch/5
  Netinput/1 -> Pattern Recognition Neural Network/1(Input)
  [nnoutpu] -> Multiport Switch/1
  VcalarmTrue1/1 -> IC1/1
  Multiport Switch/1 -> Scope3/1, MATLAB Function/1(u)
  iLalarmTrue/1 -> IC/1
  IC/1 -> MATLAB Function/2(iLAlarm), Scope/1
  IC1/1 -> MATLAB Function/3(VcAlarm), Scope1/1
  MATLAB Function/1(y) -> Scope2/1, faulType/1

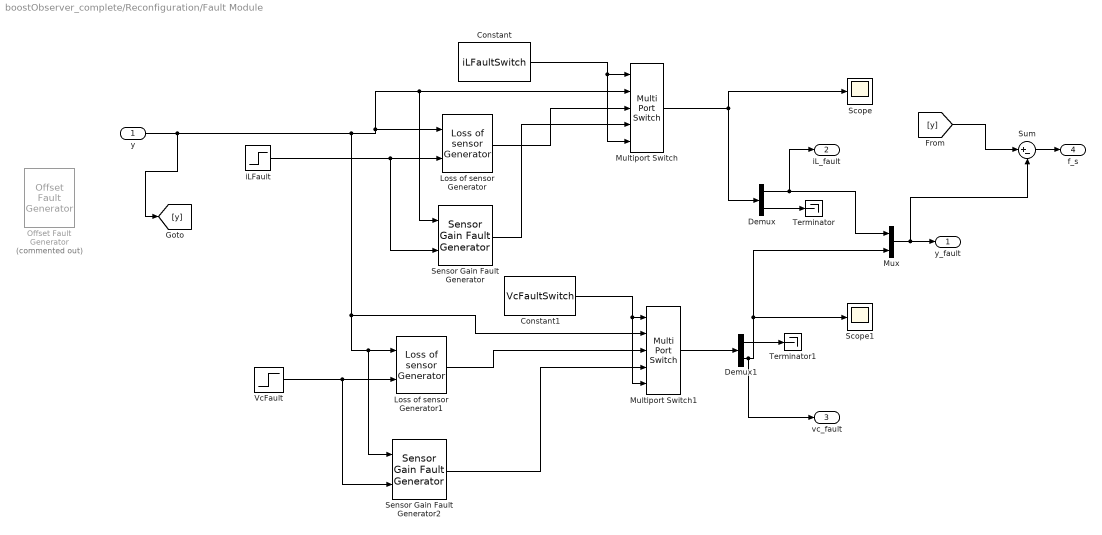
== system boostObserver_complete/Reconfiguration/Fault Module ==
  y : Inport
  Constant : Constant  Value=iLFaultSwitch
  Constant1 : Constant  Value=VcFaultSwitch
  Demux : Demux  Outputs=2
  Demux1 : Demux  Outputs=2
  Loss of sensor Generator : PhdLibrary/Loss of sensor Generator
      settings: SourceProductName=Phd Diego
  Loss of sensor Generator1 : PhdLibrary/Loss of sensor Generator
      settings: SourceProductName=Phd Diego
  Multiport Switch : MultiPortSwitch  DataPortOrder=Zero-based contiguous  DataPortForDefault=Additional data port  zeroidx=on
  Multiport Switch1 : MultiPortSwitch  DataPortOrder=Zero-based contiguous  DataPortForDefault=Additional data port  zeroidx=on
  Mux : Mux  Inputs=2
  Offset Fault Generator : PhdLibrary/Offset Fault Generator  Commented=on  s1gain=20  s2gain=20
      settings: SourceProductName=Phd Diego
  Scope : Scope
  Scope1 : Scope
  Sensor Gain Fault Generator : PhdLibrary/Sensor Gain Fault Generator  s1gain=iLGainFaultFactor  s2gain=VcGainFaultFactor
      settings: SourceProductName=Phd Diego
  Sensor Gain Fault Generator2 : PhdLibrary/Sensor Gain Fault Generator  s1gain=iLGainFaultFactor  s2gain=VcGainFaultFactor
      settings: SourceProductName=Phd Diego
  Sum : Sum  Inputs=|+-
  Terminator : Terminator
  Terminator1 : Terminator
  VcFault : Step  Time=VcFaultTime  After=2  SampleTime=0
  iLFault : Step  Time=iLFaultTime  SampleTime=0
  y_fault : Outport
  iL_fault : Outport  Port=2
  vc_fault : Outport  Port=3
  f_s : Outport  Port=4
  wires:
  iLFault/1 -> Sensor Gain Fault Generator/2, Loss of sensor Generator/2
  y/1 -> [y], Multiport Switch1/2, Sensor Gain Fault Generator2/1, Loss of sensor Generator1/1, Sensor Gain Fault Generator/1, Multiport Switch/2, Loss of sensor Generator/1
  VcFault/1 -> Sensor Gain Fault Generator2/2, Loss of sensor Generator1/2
  Constant/1 -> Multiport Switch/5, Multiport Switch/1
  Constant1/1 -> Multiport Switch1/5, Multiport Switch1/1
  Multiport Switch/1 -> Demux/1, Scope/1
  Multiport Switch1/1 -> Demux1/1
  Demux/2 -> Terminator/1
  Demux/1 -> iL_fault/1, Mux/1
  Mux/1 -> Sum/2, y_fault/1
  Demux1/1 -> Terminator1/1
  Demux1/2 -> vc_fault/1, Mux/2, Scope1/1
  Loss of sensor Generator/1 -> Multiport Switch/3
  Sensor Gain Fault Generator/1 -> Multiport Switch/4
  Sensor Gain Fault Generator2/1 -> Multiport Switch1/4
  Loss of sensor Generator1/1 -> Multiport Switch1/3
  [y] -> Sum/1
  Sum/1 -> f_s/1

== system boostObserver_complete/Reconfiguration/Flawlesse Output Separator 2x1 ==
  y : Inport
  Matrizes A1 : Constant  Value=Cf2  VectorParams1D=off
  Matrizes A2 : Constant  Value=Cf1  VectorParams1D=off
  Product : Product  Multiplication=Matrix(*)
  Product1 : Product  Multiplication=Matrix(*)
  y_f1 : Outport
  y_f2 : Outport  Port=2
  wires:
  y/1 -> Product1/2, Product/2
  Matrizes A2/1 -> Product/1
  Matrizes A1/1 -> Product1/1
  Product/1 -> y_f1/1
  Product1/1 -> y_f2/1

== system boostObserver_complete/Reconfiguration/If Action Subsystem ==
  In1 : Inport
  Action Port : ActionPort  ActionPortLabel=case [ 0 ]:
  Out1 : Outport
  wires:
  In1/1 -> Out1/1

== system boostObserver_complete/Reconfiguration/If Action Subsystem1 ==
  In1 : Inport
  Action Port : ActionPort  ActionPortLabel=default:
  Out1 : Outport
  wires:
  In1/1 -> Out1/1

== system boostObserver_complete/Reconfiguration/If Action Subsystem2 ==
  y : Inport
  Action Port : ActionPort  ActionPortLabel=case [ 2 ]:
  x_hat : Outport
  wires:
  y/1 -> x_hat/1

== system boostObserver_complete/Reconfiguration/If Action Subsystem4 ==
  y : Inport
  Action Port : ActionPort  ActionPortLabel=case [ 1 ]:
  x_hat : Outport
  wires:
  y/1 -> x_hat/1

== system boostObserver_complete/Reconfiguration/Load Module ==
  Load_add_switch : PhdLibrary/Step Perturbation  SignalSwitch=LoadAddSignalSwitch  InitialMagnitude=0  InitialTime=LoadAddTime  Magnitude=1  Duration=LoadAddDuration  enabled=LoadAddSwitch
      settings: SourceProductName=Phd Diego
  Load_remove_switch : PhdLibrary/Step Perturbation  SignalSwitch=LoadRemoveSignalSwitch  InitialMagnitude=0  InitialTime=LoadRemoveTime  Magnitude=1  Duration=LoadRemoveDuration  enabled=LoadRemoveSwitch
      settings: SourceProductName=Phd Diego
  Ro_remove : Outport
  Ro_add : Outport  Port=2
  wires:
  Load_remove_switch/1 -> Ro_remove/1
  Load_add_switch/1 -> Ro_add/1

== system boostObserver_complete/Reconfiguration/Source Module ==
  Constant1 : Constant  Value=SourceAddSwitch  VectorParams1D=off
  Constant11 : Constant  Value=u
  Source_add_switch : PhdLibrary/Step Perturbation  SignalSwitch=SourceAddSignalSwitch  InitialMagnitude=0  InitialTime=SourceAddTime  Magnitude=SourceAddFactor*u  Duration=SourceAddDuration  enabled=SourceAddSwitch
      settings: SourceProductName=Phd Diego
  Source_remove_switch : PhdLibrary/Step Perturbation  SignalSwitch=SourceRemoveSignalSwitch  InitialMagnitude=0  InitialTime=SourceRemoveTime  Magnitude=-SourceRemoveFactor*u  Duration=SourceRemoveDuration  enabled=SourceRemoveSwitch
      settings: SourceProductName=Phd Diego
  Sum : Sum  Inputs=|++
  Sum1 : Sum  Inputs=|++
  Switch : Switch  Criteria=u2 > Threshold
  u_var : Outport
  wires:
  Sum1/1 -> Switch/3
  Sum/1 -> Switch/1
  Constant11/1 -> Sum1/1, Sum/1
  Switch/1 -> u_var/1
  Source_add_switch/1 -> Sum/2
  Source_remove_switch/1 -> Sum1/2
  Constant1/1 -> Switch/2

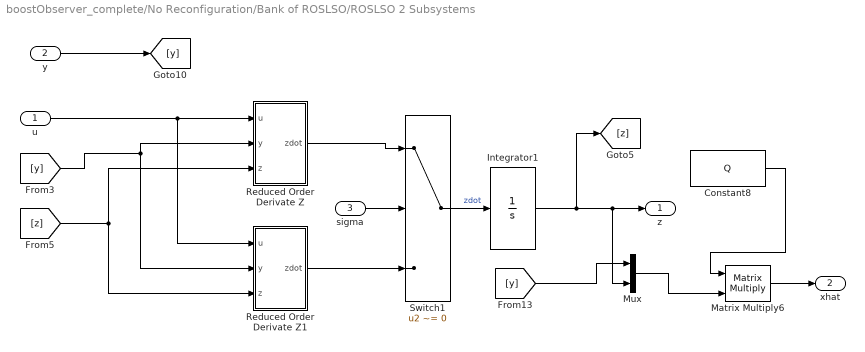
== system boostObserver_complete/No Reconfiguration/Bank of ROSLSO/ROSLSO 2 Subsystems ==
  u : Inport
  y : Inport  Port=2
  sigma : Inport  Port=3
  Constant8 : Constant  Value=Q  VectorParams1D=off
  Integrator1 : Integrator  InitialCondition=z0
  Matrix Multiply6 : Product  Multiplication=Matrix(*)
  Mux : Mux  Inputs=2
  Reduced Order Derivate Z : Subsystem  mask(Reduced Order Observer Derivate Z){F=F1, L=L1, T=T, B=B1}
      mask prompts: F "Observer gain matrix:"; L "Output gain matrix:"; T "Input gain matrix:"; B "Input matrix:"
      mask help: Reduced Order Observer Derivate Z generates just zdot, without feedbak
  Reduced Order Derivate Z1 : Subsystem  mask(Reduced Order Observer Derivate Z){F=F2, L=L2, T=T, B=B2}
      mask prompts: F "Observer gain matrix:"; L "Output gain matrix:"; T "Input gain matrix:"; B "Input matrix:"
      mask help: Reduced Order Observer Derivate Z generates just zdot, without feedbak
  Switch1 : Switch  Criteria=u2 ~= 0
  z : Outport
  xhat : Outport  Port=2
  wires:
  sigma/1 -> Switch1/2
  Switch1/1 -> Integrator1/1  "zdot"
  y/1 -> [y]
  Constant8/1 -> Matrix Multiply6/1
  Matrix Multiply6/1 -> xhat/1
  Mux/1 -> Matrix Multiply6/2
  [y] -> Mux/1
  Reduced Order Derivate Z/1(zdot) -> Switch1/1
  u/1 -> Reduced Order Derivate Z1/1(u), Reduced Order Derivate Z/1(u)
  [y] -> Reduced Order Derivate Z1/2(y), Reduced Order Derivate Z/2(y)
  [z] -> Reduced Order Derivate Z/3(z), Reduced Order Derivate Z1/3(z)
  Reduced Order Derivate Z1/1(zdot) -> Switch1/3
  Integrator1/1 -> z/1, Mux/2, [z]
